simulink model "req9"  (R2019a)
settings: Solver=FixedStepAuto  StartTime=0.0  StopTime=100  RelTol=1e-3
settings Model: Creator=e40014285  LastModifiedBy=e40014285
settings ConfigComp: CovEnable=on  CovScope=ReferencedModels  RecordCoverage=on  DVModelCoverageObjectives=MCDC  DVTestSuiteOptimization=Auto  DVDetectOutOfBounds=on  DVRebuildModelRepresentation=Always

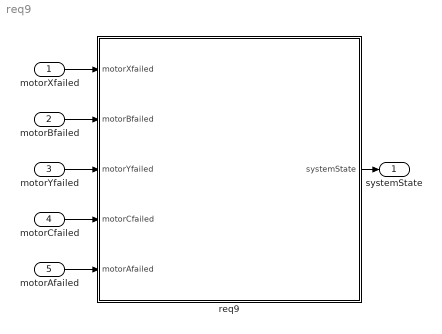
== system req9 ==
  motorXfailed : Inport
  motorBfailed : Inport  Port=2
  motorYfailed : Inport  Port=3
  motorCfailed : Inport  Port=4
  motorAfailed : Inport  Port=5
  req9 : Stateflow chart  BlockKeywords=__PRM__SERIALIZED__DATA__:Stateflow Chart,Stateflow Diagram  TreatAsAtomicUnit=on
  systemState : Outport
  wires:
  motorXfailed/1 -> req9/1(motorXfailed)
  motorBfailed/1 -> req9/2(motorBfailed)
  motorCfailed/1 -> req9/4(motorCfailed)
  motorYfailed/1 -> req9/3(motorYfailed)
  req9/1(systemState) -> systemState/1
  motorAfailed/1 -> req9/5(motorAfailed)

== stateflow chart req9/req9 ==
  state allGood
    systemState=0;
  state orangeState
    systemState=1;
  state amberState
    systemState=2;
  state redState
    systemState=3;
  (default) -> allGood
  allGood -> orangeState : [motorAfailed || motorBfailed || motorCfailed]
  orangeState -> amberState : [motorXfailed || motorYfailed]
  amberState -> redState : [motorXfailed && motorYfailed]
  data: motorXfailed input; motorBfailed input; motorYfailed input; motorCfailed input; motorAfailed input; systemState output
